simulink model "potencialaccion"  (Simulink 7.5)
settings: Solver=ode45  StartTime=0.0  StopTime=4  RelTol=1e-3
settings Model: Creator=My Laptop  LastModifiedBy=My Laptop

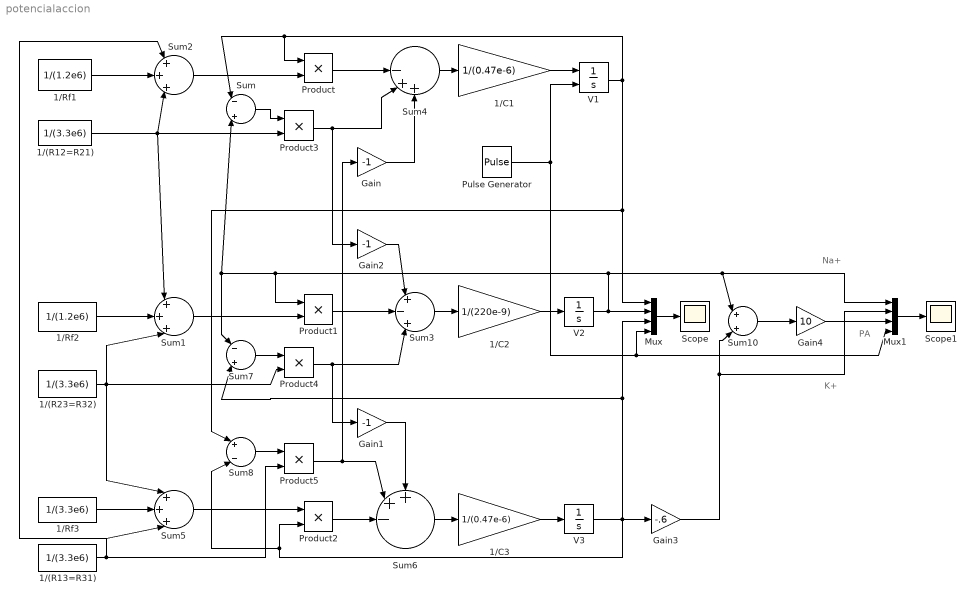
== system potencialaccion ==
  note: K+
  note: Na+
  note: PA
  1/(R12=R21) : Constant  Value=1/(3.3e6)  OutDataType=fixdt(1, 16)  OutScaling=2^0
  1/(R13=R31) : Constant  Value=1/(3.3e6)  OutDataType=fixdt(1, 16)  OutScaling=2^0
  1/(R23=R32) : Constant  Value=1/(3.3e6)  OutDataType=fixdt(1, 16)  OutScaling=2^0
  1/C1 : Gain  Gain=1/(0.47e-6)  ParameterDataType=fixdt(1, 16)  ParameterScaling=2^0  OutDataType=fixdt(1, 16)  OutScaling=2^0
  1/C2 : Gain  Gain=1/(220e-9)  ParameterDataType=fixdt(1, 16)  ParameterScaling=2^0  OutDataType=fixdt(1, 16)  OutScaling=2^0
  1/C3 : Gain  Gain=1/(0.47e-6)  ParameterDataType=fixdt(1, 16)  ParameterScaling=2^0  OutDataType=fixdt(1, 16)  OutScaling=2^0
  1/Rf1 : Constant  Value=1/(1.2e6)  OutDataType=fixdt(1, 16)  OutScaling=2^0
  1/Rf2 : Constant  Value=1/(1.2e6)  OutDataType=fixdt(1, 16)  OutScaling=2^0
  1/Rf3 : Constant  Value=1/(3.3e6)  OutDataType=fixdt(1, 16)  OutScaling=2^0
  Gain : Gain  Gain=-1  ParameterDataType=fixdt(1, 16)  ParameterScaling=2^0  OutDataType=fixdt(1, 16)  OutScaling=2^0
  Gain1 : Gain  Gain=-1  ParameterDataType=fixdt(1, 16)  ParameterScaling=2^0  OutDataType=fixdt(1, 16)  OutScaling=2^0
  Gain2 : Gain  Gain=-1  ParameterDataType=fixdt(1, 16)  ParameterScaling=2^0  OutDataType=fixdt(1, 16)  OutScaling=2^0
  Gain3 : Gain  Gain=-.6  ParameterDataType=fixdt(1, 16)  ParameterScaling=2^0  OutDataType=fixdt(1, 16)  OutScaling=2^0
  Gain4 : Gain  Gain=10  ParameterDataType=fixdt(1, 16)  ParameterScaling=2^0  OutDataType=fixdt(1, 16)  OutScaling=2^0
  Mux : Mux
  Mux1 : Mux
  Product{,1..5} (6 alike) : Product  OutDataType=fixdt(1, 16)  OutScaling=2^0  RndMeth=Zero
  Pulse Generator : DiscretePulseGenerator  PulseType=Time based  Amplitude=1  Period=4  PulseWidth=1  PhaseDelay=0  SampleTime=1
  Scope : Scope
      settings: TimeRange=1000  YMin=-0.2  YMax=1.2
  Scope1 : Scope
      settings: TimeRange=1000  YMin=-0.2  YMax=1.2
  Sum : Sum  Inputs=|-|+|  OutDataType=fixdt(1, 16)  OutScaling=2^0
  Sum1 : Sum  Inputs=|+|+|+|  OutDataType=fixdt(1, 16)  OutScaling=2^0
  Sum10 : Sum  Inputs=|+|+|  OutDataType=fixdt(1, 16)  OutScaling=2^0
  Sum2 : Sum  Inputs=|+|+|+|  OutDataType=fixdt(1, 16)  OutScaling=2^0
  Sum3 : Sum  Inputs=|+|-|+|  OutDataType=fixdt(1, 16)  OutScaling=2^0
  Sum4 : Sum  Inputs=||||-|+|+  OutDataType=fixdt(1, 16)  OutScaling=2^0
  Sum5 : Sum  Inputs=|+|+|+|  OutDataType=fixdt(1, 16)  OutScaling=2^0
  Sum6 : Sum  Inputs=+|+|-||||  OutDataType=fixdt(1, 16)  OutScaling=2^0
  Sum7 : Sum  Inputs=|-|+|  OutDataType=fixdt(1, 16)  OutScaling=2^0
  Sum8 : Sum  Inputs=|+|-|  OutDataType=fixdt(1, 16)  OutScaling=2^0
  V1 : Integrator  ExternalReset=level  InitialCondition=5
  V2 : Integrator
  V3 : Integrator
  wires:
  1/C1/1 -> V1/1
  1/C2/1 -> V2/1
  1/C3/1 -> V3/1
  Mux/1 -> Scope/1
  V1/1 -> Mux/1, Sum8/1, Product/1, Sum/1
  V2/1 -> Mux/2, Product1/1, Sum7/1, Sum/2, Sum10/1, Mux1/1
  V3/1 -> Product2/2, Sum8/2, Mux/3, Sum7/2, Gain3/1
  Sum3/1 -> 1/C2/1
  Sum4/1 -> 1/C1/1
  Sum6/1 -> 1/C3/1
  Product1/1 -> Sum3/2
  Sum2/1 -> Product/2
  Sum1/1 -> Product1/2
  Sum5/1 -> Product2/1
  1/Rf1/1 -> Sum2/2
  1/Rf2/1 -> Sum1/2
  1/Rf3/1 -> Sum5/2
  1/(R13=R31)/1 -> Sum5/3, Sum2/1, Product5/2
  1/(R23=R32)/1 -> Sum5/1, Sum1/3, Product4/2
  1/(R12=R21)/1 -> Sum2/3, Sum1/1, Product3/2
  Product/1 -> Sum4/1
  Product3/1 -> Sum4/2, Gain2/1
  Product2/1 -> Sum6/3
  Product5/1 -> Sum6/2, Gain/1
  Gain/1 -> Sum4/3
  Gain1/1 -> Sum6/1
  Product4/1 -> Sum3/3, Gain1/1
  Gain2/1 -> Sum3/1
  Sum/1 -> Product3/1
  Sum7/1 -> Product4/1
  Sum8/1 -> Product5/1
  Pulse Generator/1 -> V1/2, Mux/4, Mux1/4
  Mux1/1 -> Scope1/1
  Gain3/1 -> Sum10/2, Mux1/2
  Gain4/1 -> Mux1/3
  Sum10/1 -> Gain4/1
